simulink model "omnibundle"  (R2018b)
settings: Solver=ode2  StartTime=0.0  StopTime=40  FixedStep=0.01  RelTol=1e-3
values from neighbouring files (symbols this model uses):
  dq0 = [1 0 0]'    [main.m]
  q0 = [0 0 0]'    [main.m]
settings Model: Creator=Renata  LastModifiedBy=lucas

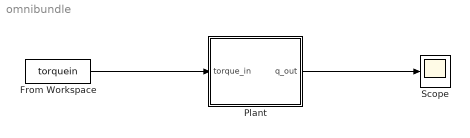
== system omnibundle ==
  From Workspace : FromWorkspace  VariableName=torquein  SampleTime=0
  Plant : Subsystem
  Scope : Scope
  wires:
  From Workspace/1 -> Plant/1(torque_in)
  Plant/1(q_out) -> Scope/1

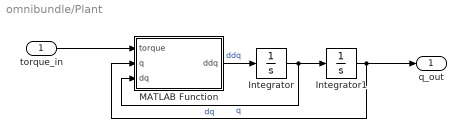
== system omnibundle/Plant ==
  torque_in : Inport
  Integrator : Integrator  InitialCondition=dq0
  Integrator1 : Integrator  InitialCondition=q0
  MATLAB Function : MATLAB Function  TreatAsAtomicUnit=on
  q_out : Outport
  wires:
  MATLAB Function/1(ddq) -> Integrator/1  "ddq"
  Integrator/1 -> MATLAB Function/3(dq), Integrator1/1  "dq"
  torque_in/1 -> MATLAB Function/1(torque)
  Integrator1/1 -> q_out/1, MATLAB Function/2(q)  "q"

== matlab function omnibundle/Plant/MATLAB Function ==
  data: torque input; q input; dq input; ddq output
function ddq = fcn(torque,q,dq)
    
    ddq = dyn_omni_bundle_fun(9.8, q, dq, torque);
